simulink subsystem "startSkew"  (R2021a)
settings: Solver=VariableStepAuto  StartTime=0.0  StopTime=10.0  RelTol=1e-3
libraries: sharedutil x1
settings Model: Creator=noraw  LastModifiedBy=noraw

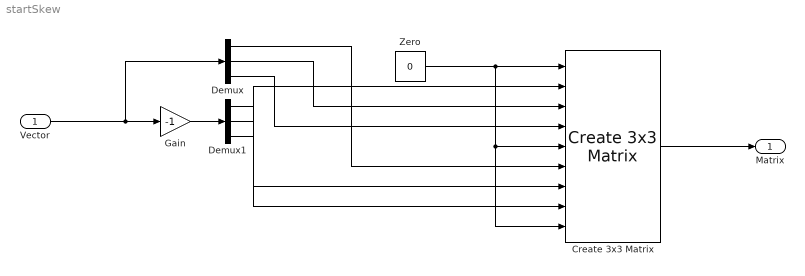
== system startSkew ==
  Vector : Inport
  Create 3x3 Matrix : sharedutil/Create 3x3 Matrix  aMode=aMode
      settings: SourceProductBaseCode=AE,PW,MT,UV,VE,VP
  Demux : Demux  Outputs=3
  Demux1 : Demux  Outputs=3
  Gain : Gain  Gain=-1
  Zero : Constant  Value=0  OutDataTypeStr=Inherit: Inherit via back propagation
  Matrix : Outport  PortDimensions=[3 3]
  wires:
  Gain/1 -> Demux1/1
  Demux/1 -> Create 3x3 Matrix/6
  Demux1/2 -> Create 3x3 Matrix/7
  Vector/1 -> Demux/1, Gain/1
  Demux1/1 -> Create 3x3 Matrix/8
  Demux1/3 -> Create 3x3 Matrix/2
  Zero/1 -> Create 3x3 Matrix/1, Create 3x3 Matrix/5, Create 3x3 Matrix/9
  Demux/3 -> Create 3x3 Matrix/4
  Demux/2 -> Create 3x3 Matrix/3
  Create 3x3 Matrix/1 -> Matrix/1
